simulink model "Q_1_A"  (R2020a)
settings: Solver=VariableStepAuto  StartTime=0.0  StopTime=10.0  RelTol=1e-3
settings Model: Creator=Admin  LastModifiedBy=Admin

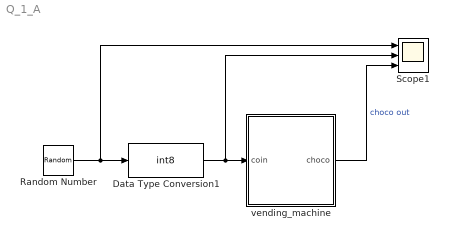
== system Q_1_A ==
  Data Type Conversion1 : DataTypeConversion  OutDataTypeStr=int8  RndMeth=Nearest
  Random Number : RandomNumber  Variance=2  Seed=337  SampleTime=10
  Scope1 : Scope  NumInputPorts=3
  vending_machine : Stateflow chart  TreatAsAtomicUnit=on
  wires:
  Random Number/1 -> Scope1/1, Data Type Conversion1/1
  Data Type Conversion1/1 -> Scope1/2, vending_machine/1(coin)
  vending_machine/1(choco) -> Scope1/3  "choco out"

== stateflow chart Q_1_A/vending_machine ==
  settings: stateMachineType=MEALY_MACHINE  initializeOutput=1
  state Twenty_five_paise
  state No_paise
  state Fifty_paise
  state One_rupee
  No_paise -> Twenty_five_paise [order 1] : [coin==1]{choco=0}
  Twenty_five_paise -> No_paise [order 2] : [coin==3]{choco=1}
  Twenty_five_paise -> One_rupee [order 1] : [coin==1]{choco=0}
  One_rupee -> Twenty_five_paise [order 3] : [coin==3]{choco=1}
  (default) -> No_paise
  No_paise -> Fifty_paise [order 2] : [coin==2]{choco=0}
  Fifty_paise -> No_paise [order 2] : [coin==3]{choco=1}
  One_rupee -> No_paise [order 1] : [coin==2 || coin==1]{choco=1}
  No_paise -> One_rupee [order 3] : [coin==3]{choco=0}
  Fifty_paise -> One_rupee [order 1] : [coin==2]{choco=0}
  One_rupee -> Fifty_paise [order 2] : [coin==3]{choco=1}
  data: coin input int8; choco output double
